simulink library "inp"  (Simulink 7.4)
settings: Solver=ode45  StartTime=0.0  StopTime=10.0  RelTol=1e-3
undefined symbols (not defined in the file): AINP_BrkPedalInterp_X_bar, C_TASK_10MS_S, ENUM_SHIFTER_D, ENUM_SHIFTER_N, ENUM_SHIFTER_P, ENUM_SHIFTER_R, KINP_BonnetCloseVehSpdThre_kph, KINP_EDUCoolantTempFilTm_s, KINP_EDUOilPressureFilTm_s, KINP_EDUOilTempFilTm_s, KINP_EDUSynchDisp_mm, KINP_EDUSynchPosnPWMDC_pct_LowerLimit, KINP_EDUSynchPosnPWMDC_pct_ovrdflg, KINP_EDUSynchPosnPWMDC_pct_ovrdval, KINP_EDUSynchPosnPWMDC_pct_UpperLimit, KINP_ShifterPosConfirmD_s, KINP_ShifterPosConfirmN_s, KINP_ShifterPosConfirmP_s, KINP_ShifterPosConfirmR_s, KINP_SingleAccPedalFltRateLim_pct, KINP_TMSpd2VehSpdSigNeg_rpm, KINP_TMSpd2VehSpdSigPos_rpm, KINP_ValidCheck_EDUSynchPosnPWMDC_dec, KINP_ValidCheck_EDUSynchPosnPWMDC_inc, KINP_ValidCheck_EDUSynchPosnPWMDC_lim, KINP_VehSpdSigKeepThres_kph, KPH2MPS, MIN2SEC, MINP_BrkPedalInterp_pct, MPS2KPH, PI, seat_version_control_block_callbacks, TIRE_RADIUS
libraries: inp_lib x166, hcu_lib x4, simulink x1
(part 8 of 9)

== system inp/INP/INP_50MS/BSRV_in_ovrdvals ==
  Constant: VSRV_AmbientTempIn_C_ovrdval : Constant  Value=0.0  OutDataTypeMode=single  OutDataTypeStr=single
  Constant: VSRV_AmbientTempValidIn_flg_ovrdval : Constant  Value=0  OutDataTypeMode=boolean  OutDataTypeStr=boolean
  Constant: VSRV_BMSCellTempMinIn_C_ovrdval : Constant  Value=0  OutDataTypeMode=boolean  OutDataTypeStr=boolean
  Constant: VSRV_BMSCellTempMinValidIn_flg_ovrdval : Constant  Value=0  OutDataTypeMode=boolean  OutDataTypeStr=boolean
  Constant: VSRV_BMSColdCrkCtrlIn_enum_ovrdval : Constant  Value=0  OutDataTypeMode=boolean  OutDataTypeStr=boolean
  Constant: VSRV_BMSHSC2FrP01Active_flg_ovrdval : Constant  Value=0  OutDataTypeMode=boolean  OutDataTypeStr=boolean
  Constant: VSRV_BMSHSC2FrP01ProtFault_flg_ovrdval : Constant  Value=0  OutDataTypeMode=boolean  OutDataTypeStr=boolean
  Constant: VSRV_BMSHSC2FrP02Active_flg_ovrdval : Constant  Value=0  OutDataTypeMode=boolean  OutDataTypeStr=boolean
  Constant: VSRV_BMSHSC2FrP02ProtFault_flg_ovrdval : Constant  Value=0  OutDataTypeMode=boolean  OutDataTypeStr=boolean
  Constant: VSRV_BMSMainRelayStatIn_enum_ovrdval : Constant  Value=0  OutDataTypeMode=uint8  OutDataTypeStr=uint8
  Constant: VSRV_BMSPackSOCDispIn_pct_ovrdval : Constant  Value=0  OutDataTypeMode=boolean  OutDataTypeStr=boolean
  Constant: VSRV_BMSPackSOCDispValidIn_pct_ovrdval : Constant  Value=0  OutDataTypeMode=boolean  OutDataTypeStr=boolean
  Constant: VSRV_HVBattBasicStatusIn_enum_ovrdval : Constant  Value=0  OutDataTypeMode=uint8  OutDataTypeStr=uint8
  Constant: VSRV_HVBattCellTempMaxIn_C_ovrdval : Constant  Value=0.0  OutDataTypeMode=single  OutDataTypeStr=single
  Constant: VSRV_HVBattCellTempMaxValidIn_flg_ovrdval : Constant  Value=0  OutDataTypeMode=boolean  OutDataTypeStr=boolean
  Constant: VSRV_HVBattChargerPluggedIn_flg_ovrdval : Constant  Value=0  OutDataTypeMode=boolean  OutDataTypeStr=boolean
  Constant: VSRV_HVBattChillerOffReqIn_flg_ovrdval : Constant  Value=0  OutDataTypeMode=boolean  OutDataTypeStr=boolean
  Constant: VSRV_HVBattCoolantTempIn_C_ovrdval : Constant  Value=0.0  OutDataTypeMode=single  OutDataTypeStr=single
  Constant: VSRV_HVBattCoolantTempValidIn_flg_ovrdval : Constant  Value=0  OutDataTypeMode=boolean  OutDataTypeStr=boolean
  Constant: VSRV_HVBattCoolingPumpStatusIn_enum_ovrdval : Constant  Value=0  OutDataTypeMode=uint8  OutDataTypeStr=uint8
  Constant: VSRV_HVBattCurrentIn_A_ovrdval : Constant  Value=0.0  OutDataTypeMode=single  OutDataTypeStr=single
  Constant: VSRV_HVBattCurrentValidIn_flg_ovrdval : Constant  Value=0  OutDataTypeMode=boolean  OutDataTypeStr=boolean
  Constant: VSRV_HVBattHVILClosedIn_flg_ovrdval : Constant  Value=0  OutDataTypeMode=boolean  OutDataTypeStr=boolean
  Constant: VSRV_HVBattIsolationResistanceIn_kohm_ovrdval : Constant  Value=0.0  OutDataTypeMode=single  OutDataTypeStr=single
  Constant: VSRV_HVBattIsolationResistanceValidIn_flg_ovrdval : Constant  Value=0  OutDataTypeMode=boolean  OutDataTypeStr=boolean
  Constant: VSRV_HVBattSOCIn_pct_ovrdval : Constant  Value=0.0  OutDataTypeMode=single  OutDataTypeStr=single
  Constant: VSRV_HVBattSOCValidIn_flg_ovrdval : Constant  Value=0  OutDataTypeMode=boolean  OutDataTypeStr=boolean
  Constant: VSRV_HVBattVoltageIn_V_ovrdval : Constant  Value=0.0  OutDataTypeMode=single  OutDataTypeStr=single
  Constant: VSRV_HVBattVoltageValidIn_flg_ovrdval : Constant  Value=0  OutDataTypeMode=boolean  OutDataTypeStr=boolean
  Constant: VSRV_KeySwitchStateCRKIn_flg_ovrdval : Constant  Value=0  OutDataTypeMode=boolean  OutDataTypeStr=boolean
  Constant: VSRV_SMUHSCFrP00Active_flg_ovrdval : Constant  Value=0  OutDataTypeMode=boolean  OutDataTypeStr=boolean
  Constant: VSRV_SMUHSCFrP03Active_flg_ovrdval : Constant  Value=0  OutDataTypeMode=boolean  OutDataTypeStr=boolean
  Constant: VSRV_SMUHSCFrP08Active_flg_ovrdval : Constant  Value=0  OutDataTypeMode=boolean  OutDataTypeStr=boolean
  inputs_bus : BusCreator  Inputs=33
  output_bus : Outport
  wires:
  Constant: VSRV_BMSPackSOCDispValidIn_pct_ovrdval/1 -> inputs_bus/33  "VSRV_BMSPackSOCDispValidIn_pct_ovrdval"
  Constant: VSRV_BMSPackSOCDispIn_pct_ovrdval/1 -> inputs_bus/32  "VSRV_BMSPackSOCDispIn_pct_ovrdval"
  Constant: VSRV_BMSCellTempMinValidIn_flg_ovrdval/1 -> inputs_bus/31  "VSRV_BMSCellTempMinValidIn_flg_ovrdval"
  Constant: VSRV_BMSCellTempMinIn_C_ovrdval/1 -> inputs_bus/30  "VSRV_BMSCellTempMinIn_C_ovrdval"
  Constant: VSRV_BMSColdCrkCtrlIn_enum_ovrdval/1 -> inputs_bus/29  "VSRV_BMSColdCrkCtrlIn_enum_ovrdval"
  Constant: VSRV_SMUHSCFrP00Active_flg_ovrdval/1 -> inputs_bus/28  "VSRV_SMUHSCFrP00Active_flg_ovrdval"
  Constant: VSRV_HVBattIsolationResistanceValidIn_flg_ovrdval/1 -> inputs_bus/27  "VSRV_HVBattIsolationResistanceValidIn_flg_ovrdval"
  Constant: VSRV_HVBattIsolationResistanceIn_kohm_ovrdval/1 -> inputs_bus/26  "VSRV_HVBattIsolationResistanceIn_kohm_ovrdval"
  Constant: VSRV_SMUHSCFrP08Active_flg_ovrdval/1 -> inputs_bus/25  "VSRV_SMUHSCFrP08Active_flg_ovrdval"
  Constant: VSRV_SMUHSCFrP03Active_flg_ovrdval/1 -> inputs_bus/24  "VSRV_SMUHSCFrP03Active_flg_ovrdval"
  Constant: VSRV_KeySwitchStateCRKIn_flg_ovrdval/1 -> inputs_bus/23  "VSRV_KeySwitchStateCRKIn_flg_ovrdval"
  Constant: VSRV_HVBattVoltageValidIn_flg_ovrdval/1 -> inputs_bus/22  "VSRV_HVBattVoltageValidIn_flg_ovrdval"
  Constant: VSRV_HVBattVoltageIn_V_ovrdval/1 -> inputs_bus/21  "VSRV_HVBattVoltageIn_V_ovrdval"
  Constant: VSRV_HVBattSOCValidIn_flg_ovrdval/1 -> inputs_bus/20  "VSRV_HVBattSOCValidIn_flg_ovrdval"
  Constant: VSRV_HVBattSOCIn_pct_ovrdval/1 -> inputs_bus/19  "VSRV_HVBattSOCIn_pct_ovrdval"
  Constant: VSRV_HVBattBasicStatusIn_enum_ovrdval/1 -> inputs_bus/18  "VSRV_HVBattBasicStatusIn_enum_ovrdval"
  Constant: VSRV_HVBattHVILClosedIn_flg_ovrdval/1 -> inputs_bus/17  "VSRV_HVBattHVILClosedIn_flg_ovrdval"
  Constant: VSRV_HVBattCurrentValidIn_flg_ovrdval/1 -> inputs_bus/16  "VSRV_HVBattCurrentValidIn_flg_ovrdval"
  Constant: VSRV_HVBattCurrentIn_A_ovrdval/1 -> inputs_bus/15  "VSRV_HVBattCurrentIn_A_ovrdval"
  Constant: VSRV_HVBattCoolingPumpStatusIn_enum_ovrdval/1 -> inputs_bus/14  "VSRV_HVBattCoolingPumpStatusIn_enum_ovrdval"
  Constant: VSRV_HVBattCoolantTempValidIn_flg_ovrdval/1 -> inputs_bus/13  "VSRV_HVBattCoolantTempValidIn_flg_ovrdval"
  Constant: VSRV_HVBattCoolantTempIn_C_ovrdval/1 -> inputs_bus/12  "VSRV_HVBattCoolantTempIn_C_ovrdval"
  Constant: VSRV_HVBattChillerOffReqIn_flg_ovrdval/1 -> inputs_bus/11  "VSRV_HVBattChillerOffReqIn_flg_ovrdval"
  Constant: VSRV_HVBattChargerPluggedIn_flg_ovrdval/1 -> inputs_bus/10  "VSRV_HVBattChargerPluggedIn_flg_ovrdval"
  Constant: VSRV_HVBattCellTempMaxValidIn_flg_ovrdval/1 -> inputs_bus/9  "VSRV_HVBattCellTempMaxValidIn_flg_ovrdval"
  Constant: VSRV_HVBattCellTempMaxIn_C_ovrdval/1 -> inputs_bus/8  "VSRV_HVBattCellTempMaxIn_C_ovrdval"
  Constant: VSRV_BMSMainRelayStatIn_enum_ovrdval/1 -> inputs_bus/7  "VSRV_BMSMainRelayStatIn_enum_ovrdval"
  Constant: VSRV_BMSHSC2FrP02Active_flg_ovrdval/1 -> inputs_bus/6  "VSRV_BMSHSC2FrP02Active_flg_ovrdval"
  Constant: VSRV_BMSHSC2FrP01Active_flg_ovrdval/1 -> inputs_bus/5  "VSRV_BMSHSC2FrP01Active_flg_ovrdval"
  Constant: VSRV_AmbientTempValidIn_flg_ovrdval/1 -> inputs_bus/4  "VSRV_AmbientTempValidIn_flg_ovrdval"
  Constant: VSRV_AmbientTempIn_C_ovrdval/1 -> inputs_bus/3  "VSRV_AmbientTempIn_C_ovrdval"
  Constant: VSRV_BMSHSC2FrP02ProtFault_flg_ovrdval/1 -> inputs_bus/2  "VSRV_BMSHSC2FrP02ProtFault_flg_ovrdval"
  Constant: VSRV_BMSHSC2FrP01ProtFault_flg_ovrdval/1 -> inputs_bus/1  "VSRV_BMSHSC2FrP01ProtFault_flg_ovrdval"
  inputs_bus/1 -> output_bus/1  "output_bus_ovrdval"

== system inp/INP/INP_50MS/Message (50ms) BMS_HSC2_FrP01 ==
  BHAL_IN_50ms : Inport
  BSRV_In_ovrdflgs : Inport  Port=2
  BSRV_In_ovrdvals : Inport  Port=3
  VINP_BMSMsgAlive_flg : Inport  Port=4
  Bus Creator : BusCreator  Inputs=5
  Bus Selector1 : BusSelector  OutputSignals=VHAL_HVBattSOCValidIn_flg
  Bus Selector11 : BusSelector  OutputSignals=VSRV_HVBattCurrentIn_A_ovrdval
  Bus Selector118 : BusSelector  OutputSignals=VHAL_HVBattSOCIn_pct
  Bus Selector120 : BusSelector  OutputSignals=VSRV_HVBattSOCIn_pct_ovrdflg
  Bus Selector142 : BusSelector  OutputSignals=VSRV_HVBattVoltageIn_V_ovrdflg
  Bus Selector143 : BusSelector  OutputSignals=VSRV_HVBattVoltageIn_V_ovrdval
  Bus Selector144 : BusSelector  OutputSignals=VHAL_HVBattVoltageIn_V
  Bus Selector15 : BusSelector  OutputSignals=VHAL_HVBattCurrentIn_A
  Bus Selector19 : BusSelector  OutputSignals=VSRV_HVBattCurrentIn_A_ovrdflg
  Bus Selector2 : BusSelector  OutputSignals=VSRV_BMSHSC2FrP01Active_flg_ovrdflg
  Bus Selector22 : BusSelector  OutputSignals=VHAL_HVBattCurrentValidIn_flg
  Bus Selector28 : BusSelector  OutputSignals=VSRV_HVBattSOCIn_pct_ovrdval
  Bus Selector3 : BusSelector  OutputSignals=VSRV_BMSHSC2FrP01Active_flg_ovrdval
  Bus Selector31 : BusSelector  OutputSignals=VSRV_HVBattIsolationResistanceIn_kohm_ovrdval
  Bus Selector32 : BusSelector  OutputSignals=VHAL_HVBattIsolationResistanceIn_kohm
  Bus Selector34 : BusSelector  OutputSignals=VSRV_HVBattIsolationResistanceIn_kohm_ovrdflg
  Bus Selector4 : BusSelector  OutputSignals=VHAL_HVBattVoltageValidIn_flg
  Bus Selector5 : BusSelector  OutputSignals=VHAL_HVBattIsolationResistanceValidIn_flg
  Subsys VINP_BMSHSC2FrP01Active_flg : inp_lib/override  SystemSampleTime=-1  cal_ovrdflg=KINP_BMSHSC2FrP01Active_ovrdflg  cal_ovrdval=KINP_BMSHSC2FrP01Active_flg_ovrdval
  Subsys VINP_HVBattCurrent_A : inp_lib/valid_msgactv_sat_ovrd  SystemSampleTime=-1  cal_ovrdflg=KINP_HVBattCurrent_A_ovrdflg  cal_ovrdval=KINP_HVBattCurrent_A_ovrdval  lim=KINP_ValidCheck_HVBattCurrent_lim  inc=KINP_ValidCheck_HVBattCurrent_inc  dec=KINP_ValidCheck_HVBattCurrent_dec  default=KINP_HVBattCurrentDefault_A  hi=KINP_HVBattCurrent_A_Max  lo=KINP_HVBattCurrent_A_Min
  Subsys VINP_HVBattIsolationResistance_kohm : inp_lib/valid_msgactv_sat_ovrd  SystemSampleTime=-1  cal_ovrdflg=KINP_HVBattIsolationResistance_kohm_ovrdflg  cal_ovrdval=KINP_HVBattIsolationResistance_kohm_ovrdval  lim=KINP_ValidCheck_HVBattIsolationResistance_lim  inc=KINP_ValidCheck_HVBattIsolationResistance_inc  dec=KINP_ValidCheck_HVBattIsolationResistance_dec  default=KINP_HVBattIsolationResistanceDefault_kohm  hi=KINP_HVBattIsolationResistance_kohm_Max  lo=KINP_HVBattIsolationResistance_kohm_Min
  Subsys VINP_HVBattSOC_pct : inp_lib/valid_msgactv_sat_ovrd  SystemSampleTime=-1  cal_ovrdflg=KINP_HVBattSOC_pct_ovrdflg  cal_ovrdval=KINP_HVBattSOC_pct_ovrdval  lim=KINP_ValidCheck_HVBattSOC_lim  inc=KINP_ValidCheck_HVBattSOC_inc  dec=KINP_ValidCheck_HVBattSOC_dec  default=KINP_HVBattSOCDefault_pct  hi=KINP_HVBattSOC_pct_Max  lo=KINP_HVBattSOC_pct_Min
  Subsys VINP_HVBattVoltage_V : inp_lib/valid_msgactv_sat_ovrd  SystemSampleTime=-1  cal_ovrdflg=KINP_HVBattVoltage_V_ovrdflg  cal_ovrdval=KINP_HVBattVoltage_V_ovrdval  lim=KINP_ValidCheck_HVBattVoltage_lim  inc=KINP_ValidCheck_HVBattVoltage_inc  dec=KINP_ValidCheck_HVBattVoltage_dec  default=KINP_HVBattVoltageDefault_V  hi=KINP_HVBattVoltage_V_Max  lo=KINP_HVBattVoltage_V_Min
  Terminator{,1..3} (4 alike) : Terminator
  BINP_BMS_FrP01 : Outport
  wires:
  [BSRV_In_ovrdvals] -> Bus Selector3/1
  [BSRV_In_ovrdflgs] -> Bus Selector2/1
  Bus Creator/1 -> BINP_BMS_FrP01/1  "BINP_BMS_FrP01"
  BSRV_In_ovrdvals/1 -> [BSRV_In_ovrdvals]
  BSRV_In_ovrdflgs/1 -> [BSRV_In_ovrdflgs]
  VINP_BMSMsgAlive_flg/1 -> [VINP_BMSMsgAlive_flg]
  [BSRV_In_ovrdflgs] -> Bus Selector120/1
  [BSRV_In_ovrdvals] -> Bus Selector28/1
  [BSRV_In_ovrdflgs] -> Bus Selector142/1
  [BSRV_In_ovrdvals] -> Bus Selector143/1
  [BSRV_In_ovrdflgs] -> Bus Selector19/1
  [BSRV_In_ovrdvals] -> Bus Selector11/1
  [BSRV_In_ovrdflgs] -> Bus Selector34/1
  [BSRV_In_ovrdvals] -> Bus Selector31/1
  BHAL_IN_50ms/1 -> Bus Selector32/1, Bus Selector5/1, Bus Selector118/1, Bus Selector1/1, Bus Selector4/1, Bus Selector22/1, Bus Selector15/1, Bus Selector144/1
  Bus Selector2/1 -> Subsys VINP_BMSHSC2FrP01Active_flg/2  "<VSRV_BMSHSC2FrP01Active_flg_ovrdflg>"
  Bus Selector3/1 -> Subsys VINP_BMSHSC2FrP01Active_flg/3  "<VSRV_BMSHSC2FrP01Active_flg_ovrdval>"
  Subsys VINP_BMSHSC2FrP01Active_flg/1 -> Bus Creator/5  "VINP_BMSHSC2FrP01Active_flg"
  Bus Selector15/1 -> Subsys VINP_HVBattCurrent_A/1  "<VHAL_HVBattCurrentIn_A>"
  Bus Selector22/1 -> Subsys VINP_HVBattCurrent_A/2  "<VHAL_HVBattCurrentValidIn_flg>"
  Bus Selector19/1 -> Subsys VINP_HVBattCurrent_A/3  "<VSRV_HVBattCurrentIn_A_ovrdflg>"
  Bus Selector11/1 -> Subsys VINP_HVBattCurrent_A/4  "<VSRV_HVBattCurrentIn_A_ovrdval>"
  [MsgAlive_flgs] -> Subsys VINP_HVBattCurrent_A/5
  Subsys VINP_HVBattCurrent_A/1 -> Bus Creator/4  "VINP_HVBattCurrent_A"
  Subsys VINP_HVBattCurrent_A/2 -> Terminator/1
  Bus Selector32/1 -> Subsys VINP_HVBattIsolationResistance_kohm/1  "<VHAL_HVBattIsolationResistanceIn_kohm>"
  Bus Selector5/1 -> Subsys VINP_HVBattIsolationResistance_kohm/2  "<VHAL_HVBattIsolationResistanceValidIn_flg>"
  Bus Selector34/1 -> Subsys VINP_HVBattIsolationResistance_kohm/3  "<VSRV_HVBattIsolationResistanceIn_kohm_ovrdflg>"
  Bus Selector31/1 -> Subsys VINP_HVBattIsolationResistance_kohm/4  "<VSRV_HVBattIsolationResistanceIn_kohm_ovrdval>"
  [MsgAlive_flgs] -> Subsys VINP_HVBattIsolationResistance_kohm/5
  Subsys VINP_HVBattIsolationResistance_kohm/1 -> Bus Creator/1  "VINP_HVBattIsolationResistance_kohm"
  Subsys VINP_HVBattIsolationResistance_kohm/2 -> Terminator1/1
  Bus Selector118/1 -> Subsys VINP_HVBattSOC_pct/1  "<VHAL_HVBattSOCIn_pct>"
  Bus Selector1/1 -> Subsys VINP_HVBattSOC_pct/2  "<VHAL_HVBattSOCValidIn_flg>"
  Bus Selector120/1 -> Subsys VINP_HVBattSOC_pct/3  "<VSRV_HVBattSOCIn_pct_ovrdflg>"
  Bus Selector28/1 -> Subsys VINP_HVBattSOC_pct/4  "<VSRV_HVBattSOCIn_pct_ovrdval>"
  [MsgAlive_flgs] -> Subsys VINP_HVBattSOC_pct/5
  Subsys VINP_HVBattSOC_pct/1 -> Bus Creator/2  "VINP_HVBattSOC_pct"
  Subsys VINP_HVBattSOC_pct/2 -> Terminator2/1
  Bus Selector144/1 -> Subsys VINP_HVBattVoltage_V/1  "<VHAL_HVBattVoltageIn_V>"
  Bus Selector4/1 -> Subsys VINP_HVBattVoltage_V/2  "<VHAL_HVBattVoltageValidIn_flg>"
  Bus Selector142/1 -> Subsys VINP_HVBattVoltage_V/3  "<VSRV_HVBattVoltageIn_V_ovrdflg>"
  Bus Selector143/1 -> Subsys VINP_HVBattVoltage_V/4  "<VSRV_HVBattVoltageIn_V_ovrdval>"
  [MsgAlive_flgs] -> Subsys VINP_HVBattVoltage_V/5
  Subsys VINP_HVBattVoltage_V/1 -> Bus Creator/3  "VINP_HVBattVoltage_V"
  Subsys VINP_HVBattVoltage_V/2 -> Terminator3/1
  [VINP_BMSMsgAlive_flg] -> Subsys VINP_BMSHSC2FrP01Active_flg/1, [MsgAlive_flgs]  "VINP_BMSMsgAlive_flg"

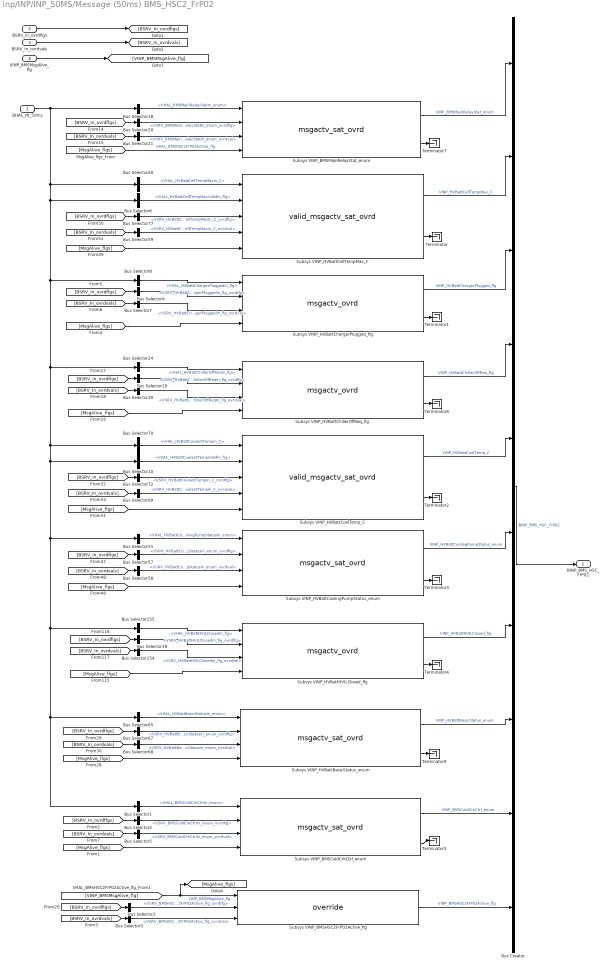
== system inp/INP/INP_50MS/Message (50ms) BMS_HSC2_FrP02 ==
  BHAL_IN_50ms : Inport
  BSRV_In_ovrdflgs : Inport  Port=2
  BSRV_In_ovrdvals : Inport  Port=3
  VINP_BMSMsgAlive_flg : Inport  Port=4
  Bus Creator : BusCreator  Inputs=10
  Bus Selector1 : BusSelector  OutputSignals=VHAL_BMSColdCrkCtrlIn_enum
  Bus Selector10 : BusSelector  OutputSignals=VHAL_HVBattCoolantTempValidIn_flg
  Bus Selector154 : BusSelector  OutputSignals=VSRV_HVBattHVILClosedIn_flg_ovrdval
  Bus Selector155 : BusSelector  OutputSignals=VHAL_HVBattHVILClosedIn_flg
  Bus Selector18 : BusSelector  OutputSignals=VHAL_BMSMainRelayStatIn_enum
  Bus Selector2 : BusSelector  OutputSignals=VSRV_BMSHSC2FrP02Active_flg_ovrdflg
  Bus Selector20 : BusSelector  OutputSignals=VSRV_BMSMainRelayStatIn_enum_ovrdflg
  Bus Selector21 : BusSelector  OutputSignals=VSRV_BMSMainRelayStatIn_enum_ovrdval
  Bus Selector24 : BusSelector  OutputSignals=VHAL_HVBattChillerOffReqIn_flg
  Bus Selector29 : BusSelector  OutputSignals=VSRV_HVBattChillerOffReqIn_flg_ovrdflg
  Bus Selector3 : BusSelector  OutputSignals=VSRV_BMSHSC2FrP02Active_flg_ovrdval
  Bus Selector30 : BusSelector  OutputSignals=VSRV_HVBattChillerOffReqIn_flg_ovrdval
  Bus Selector39 : BusSelector  OutputSignals=VSRV_HVBattHVILClosedIn_flg_ovrdflg
  Bus Selector4 : BusSelector  OutputSignals=VSRV_BMSColdCrkCtrlIn_enum_ovrdflg
  Bus Selector5 : BusSelector  OutputSignals=VSRV_BMSColdCrkCtrlIn_enum_ovrdval
  Bus Selector55 : BusSelector  OutputSignals=VHAL_HVBattCoolingPumpStatusIn_enum
  Bus Selector57 : BusSelector  OutputSignals=VSRV_HVBattCoolingPumpStatusIn_enum_ovrdflg
  Bus Selector58 : BusSelector  OutputSignals=VSRV_HVBattCoolingPumpStatusIn_enum_ovrdval
  Bus Selector59 : BusSelector  OutputSignals=VSRV_HVBattCellTempMaxIn_C_ovrdval
  Bus Selector6 : BusSelector  OutputSignals=VHAL_HVBattCellTempMaxValidIn_flg
  Bus Selector60 : BusSelector  OutputSignals=VHAL_HVBattCellTempMaxIn_C
  Bus Selector65 : BusSelector  OutputSignals=VHAL_HVBattBasicStatusIn_enum
  Bus Selector67 : BusSelector  OutputSignals=VSRV_HVBattBasicStatusIn_enum_ovrdflg
  Bus Selector68 : BusSelector  OutputSignals=VSRV_HVBattBasicStatusIn_enum_ovrdval
  Bus Selector69 : BusSelector  OutputSignals=VSRV_HVBattCoolantTempIn_C_ovrdval
  Bus Selector7 : BusSelector  OutputSignals=VSRV_HVBattChargerPluggedIn_flg_ovrdval
  Bus Selector70 : BusSelector  OutputSignals=VHAL_HVBattCoolantTempIn_C
  Bus Selector72 : BusSelector  OutputSignals=VSRV_HVBattCoolantTempIn_C_ovrdflg
  Bus Selector77 : BusSelector  OutputSignals=VSRV_HVBattCellTempMaxIn_C_ovrdflg
  Bus Selector8 : BusSelector  OutputSignals=VHAL_HVBattChargerPluggedIn_flg
  Bus Selector9 : BusSelector  OutputSignals=VSRV_HVBattChargerPluggedIn_flg_ovrdflg
  Subsys VINP_BMSColdCrkCtrl_enum : inp_lib/msgactv_sat_ovrd  SystemSampleTime=-1  cal_ovrdflg=KINP_BMSColdCrkCtrl_enum_ovrdflg  cal_ovrdval=KINP_BMSColdCrkCtrl_enum_ovrdval  default=KINP_BMSColdCrkCtrlDefault_enum  hi=KINP_BMSColdCrkCtrl_enum_Max  lo=KINP_BMSColdCrkCtrl_enum_Min
  Subsys VINP_BMSHSC2FrP02Active_flg : inp_lib/override  SystemSampleTime=-1  cal_ovrdflg=KINP_BMSHSC2FrP02Active_flg_ovrdflg  cal_ovrdval=KINP_BMSHSC2FrP02Active_flg_ovrdval
  Subsys VINP_BMSMainRelayStat_enum : inp_lib/msgactv_sat_ovrd  SystemSampleTime=-1  cal_ovrdflg=KINP_BMSMainRelayStat_enum_ovrdflg  cal_ovrdval=KINP_BMSMainRelayStat_enum_ovrdval  default=KINP_BMSMainRelayStatDefault_enum  hi=KINP_BMSMainRelayStat_enum_Max  lo=KINP_BMSMainRelayStat_enum_Min
  Subsys VINP_HVBattBasicStatus_enum : inp_lib/msgactv_sat_ovrd  SystemSampleTime=-1  cal_ovrdflg=KINP_HVBattBasicStatus_enum_ovrdflg  cal_ovrdval=KINP_HVBattBasicStatus_enum_ovrdval  default=KINP_HVBattBasicStatusDefault_enum  hi=KINP_HVBattBasicStatus_enum_Max  lo=KINP_HVBattBasicStatus_enum_Min
  Subsys VINP_HVBattCellTempMax_C : inp_lib/valid_msgactv_sat_ovrd  SystemSampleTime=-1  cal_ovrdflg=KINP_HVBattCellTempMax_C_ovrdflg  cal_ovrdval=KINP_HVBattCellTempMax_C_ovrdval  lim=KINP_ValidCheck_HVBattCellTempMax_lim  inc=KINP_ValidCheck_HVBattCellTempMax_inc  dec=KINP_ValidCheck_HVBattCellTempMax_dec  default=KINP_HVBattCellTempMaxDefault_C  hi=KINP_HVBattCellTempMax_C_Max  lo=KINP_HVBattCellTempMax_C_Min
  Subsys VINP_HVBattChargerPlugged_flg : inp_lib/msgactv_ovrd  SystemSampleTime=-1  cal_ovrdflg=KINP_HVBattChargerPlugged_flg_ovrdflg  cal_ovrdval=KINP_HVBattChargerPlugged_flg_ovrdval  default=KINP_HVBattChargerPluggedDefault_flg
  Subsys VINP_HVBattChillerOffReq_flg : inp_lib/msgactv_ovrd  SystemSampleTime=-1  cal_ovrdflg=KINP_HVBattChillerOffReq_flg_ovrdflg  cal_ovrdval=KINP_HVBattChillerOffReq_flg_ovrdval  default=KINP_HVBattChillerOffReqDefault_flg
  Subsys VINP_HVBattCoolTemp_C : inp_lib/valid_msgactv_sat_ovrd  SystemSampleTime=-1  cal_ovrdflg=KINP_HVBattCoolantTemp_C_ovrdflg  cal_ovrdval=KINP_HVBattCoolantTemp_C_ovrdval  lim=KINP_ValidCheck_HVBattCoolantTemp_lim  inc=KINP_ValidCheck_HVBattCoolantTemp_inc  dec=KINP_ValidCheck_HVBattCoolantTemp_dec  default=KINP_HVBattCoolantTempDefault_C  hi=KINP_HVBattCoolTemp_C_Max  lo=KINP_HVBattCoolTemp_C_Min
  Subsys VINP_HVBattCoolingPumpStatus_enum : inp_lib/msgactv_sat_ovrd  SystemSampleTime=-1  cal_ovrdflg=KINP_HVBattCoolingPumpStatus_enum_ovrdflg  cal_ovrdval=KINP_HVBattCoolingPumpStatus_enum_ovrdval  default=KINP_HVBattCoolingPumpStatusDefault_enum  hi=KINP_HVBattCoolingPumpStatus_enum_Max  lo=KINP_HVBattCoolingPumpStatus_enum_Min
  Subsys VINP_HVBattHVILClosed_flg : inp_lib/msgactv_ovrd  SystemSampleTime=-1  cal_ovrdflg=KINP_HVBattHVILClosed_flg_ovrdflg  cal_ovrdval=KINP_HVBattHVILClosed_flg_ovrdval  default=KINP_HVBattHVILClosedDefault_flg
  Terminator{,1..5,7..9} (9 alike) : Terminator
  BINP_BMS_HSC_FrP02 : Outport
  wires:
  Subsys VINP_BMSHSC2FrP02Active_flg/1 -> Bus Creator/10  "VINP_BMSHSC2FrP02Active_flg"
  [BSRV_In_ovrdflgs] -> Bus Selector4/1
  [BSRV_In_ovrdvals] -> Bus Selector5/1
  Bus Selector1/1 -> Subsys VINP_BMSColdCrkCtrl_enum/1  "<VHAL_BMSColdCrkCtrlIn_enum>"
  Bus Selector4/1 -> Subsys VINP_BMSColdCrkCtrl_enum/2  "<VSRV_BMSColdCrkCtrlIn_enum_ovrdflg>"
  Bus Selector5/1 -> Subsys VINP_BMSColdCrkCtrl_enum/3  "<VSRV_BMSColdCrkCtrlIn_enum_ovrdval>"
  [MsgAlive_flgs] -> Subsys VINP_BMSColdCrkCtrl_enum/4
  Subsys VINP_BMSColdCrkCtrl_enum/1 -> Bus Creator/9  "VINP_BMSColdCrkCtrl_enum"
  Subsys VINP_BMSColdCrkCtrl_enum/2 -> Terminator5/1
  BHAL_IN_50ms/1 -> Bus Selector60/1, Bus Selector6/1, Bus Selector8/1, Bus Selector24/1, Bus Selector70/1, Bus Selector10/1, Bus Selector55/1, Bus Selector1/1, Bus Selector65/1, Bus Selector155/1, Bus Selector18/1
  [BSRV_In_ovrdvals] -> Bus Selector21/1
  [BSRV_In_ovrdflgs] -> Bus Selector20/1
  VINP_BMSMsgAlive_flg/1 -> [VINP_BMSMsgAlive_flg]
  BSRV_In_ovrdflgs/1 -> [BSRV_In_ovrdflgs]
  BSRV_In_ovrdvals/1 -> [BSRV_In_ovrdvals]
  Bus Creator/1 -> BINP_BMS_HSC_FrP02/1  "BINP_BMS_HSC_FrP02"
  [BSRV_In_ovrdflgs] -> Bus Selector77/1
  [BSRV_In_ovrdvals] -> Bus Selector59/1
  [BSRV_In_ovrdflgs] -> Bus Selector9/1
  [BSRV_In_ovrdvals] -> Bus Selector7/1
  [BSRV_In_ovrdflgs] -> Bus Selector29/1
  [BSRV_In_ovrdvals] -> Bus Selector30/1
  [BSRV_In_ovrdflgs] -> Bus Selector72/1
  [BSRV_In_ovrdvals] -> Bus Selector69/1
  [BSRV_In_ovrdflgs] -> Bus Selector57/1
  [BSRV_In_ovrdvals] -> Bus Selector58/1
  [BSRV_In_ovrdflgs] -> Bus Selector39/1
  [BSRV_In_ovrdvals] -> Bus Selector154/1
  [BSRV_In_ovrdflgs] -> Bus Selector67/1
  [BSRV_In_ovrdvals] -> Bus Selector68/1
  [BSRV_In_ovrdvals] -> Bus Selector3/1
  [BSRV_In_ovrdflgs] -> Bus Selector2/1
  Bus Selector2/1 -> Subsys VINP_BMSHSC2FrP02Active_flg/2  "<VSRV_BMSHSC2FrP02Active_flg_ovrdflg>"
  Bus Selector3/1 -> Subsys VINP_BMSHSC2FrP02Active_flg/3  "<VSRV_BMSHSC2FrP02Active_flg_ovrdval>"
  Bus Selector60/1 -> Subsys VINP_HVBattCellTempMax_C/1  "<VHAL_HVBattCellTempMaxIn_C>"
  Bus Selector6/1 -> Subsys VINP_HVBattCellTempMax_C/2  "<VHAL_HVBattCellTempMaxValidIn_flg>"
  Bus Selector77/1 -> Subsys VINP_HVBattCellTempMax_C/3  "<VSRV_HVBattCellTempMaxIn_C_ovrdflg>"
  Bus Selector59/1 -> Subsys VINP_HVBattCellTempMax_C/4  "<VSRV_HVBattCellTempMaxIn_C_ovrdval>"
  [MsgAlive_flgs] -> Subsys VINP_HVBattCellTempMax_C/5
  Subsys VINP_HVBattCellTempMax_C/1 -> Bus Creator/2  "VINP_HVBattCellTempMax_C"
  Subsys VINP_HVBattCellTempMax_C/2 -> Terminator/1
  Bus Selector8/1 -> Subsys VINP_HVBattChargerPlugged_flg/1  "<VHAL_HVBattChargerPluggedIn_flg>"
  Bus Selector9/1 -> Subsys VINP_HVBattChargerPlugged_flg/2  "<VSRV_HVBattChargerPluggedIn_flg_ovrdflg>"
  Bus Selector7/1 -> Subsys VINP_HVBattChargerPlugged_flg/3  "<VSRV_HVBattChargerPluggedIn_flg_ovrdval>"
  [MsgAlive_flgs] -> Subsys VINP_HVBattChargerPlugged_flg/4
  Subsys VINP_HVBattChargerPlugged_flg/1 -> Bus Creator/3  "VINP_HVBattChargerPlugged_flg"
  Subsys VINP_HVBattChargerPlugged_flg/2 -> Terminator1/1
  Bus Selector70/1 -> Subsys VINP_HVBattCoolTemp_C/1  "<VHAL_HVBattCoolantTempIn_C>"
  Bus Selector10/1 -> Subsys VINP_HVBattCoolTemp_C/2  "<VHAL_HVBattCoolantTempValidIn_flg>"
  Bus Selector72/1 -> Subsys VINP_HVBattCoolTemp_C/3  "<VSRV_HVBattCoolantTempIn_C_ovrdflg>"
  Bus Selector69/1 -> Subsys VINP_HVBattCoolTemp_C/4  "<VSRV_HVBattCoolantTempIn_C_ovrdval>"
  [MsgAlive_flgs] -> Subsys VINP_HVBattCoolTemp_C/5
  Subsys VINP_HVBattCoolTemp_C/1 -> Bus Creator/5  "VINP_HVBattCoolTemp_C"
  Subsys VINP_HVBattCoolTemp_C/2 -> Terminator2/1
  Bus Selector55/1 -> Subsys VINP_HVBattCoolingPumpStatus_enum/1  "<VHAL_HVBattCoolingPumpStatusIn_enum>"
  Bus Selector57/1 -> Subsys VINP_HVBattCoolingPumpStatus_enum/2  "<VSRV_HVBattCoolingPumpStatusIn_enum_ovrdflg>"
  Bus Selector58/1 -> Subsys VINP_HVBattCoolingPumpStatus_enum/3  "<VSRV_HVBattCoolingPumpStatusIn_enum_ovrdval>"
  [MsgAlive_flgs] -> Subsys VINP_HVBattCoolingPumpStatus_enum/4
  Subsys VINP_HVBattCoolingPumpStatus_enum/1 -> Bus Creator/6  "VINP_HVBattCoolingPumpStatus_enum"
  Subsys VINP_HVBattCoolingPumpStatus_enum/2 -> Terminator3/1
  Bus Selector155/1 -> Subsys VINP_HVBattHVILClosed_flg/1  "<VHAL_HVBattHVILClosedIn_flg>"
  Bus Selector39/1 -> Subsys VINP_HVBattHVILClosed_flg/2  "<VSRV_HVBattHVILClosedIn_flg_ovrdflg>"
  Bus Selector154/1 -> Subsys VINP_HVBattHVILClosed_flg/3  "<VSRV_HVBattHVILClosedIn_flg_ovrdval>"
  [MsgAlive_flgs] -> Subsys VINP_HVBattHVILClosed_flg/4
  Subsys VINP_HVBattHVILClosed_flg/1 -> Bus Creator/7  "VINP_HVBattHVILClosed_flg"
  Subsys VINP_HVBattHVILClosed_flg/2 -> Terminator4/1
  Bus Selector18/1 -> Subsys VINP_BMSMainRelayStat_enum/1  "<VHAL_BMSMainRelayStatIn_enum>"
  Bus Selector20/1 -> Subsys VINP_BMSMainRelayStat_enum/2  "<VSRV_BMSMainRelayStatIn_enum_ovrdflg>"
  Bus Selector21/1 -> Subsys VINP_BMSMainRelayStat_enum/3  "<VSRV_BMSMainRelayStatIn_enum_ovrdval>"
  [MsgAlive_flgs] -> Subsys VINP_BMSMainRelayStat_enum/4  "VHAL_BMSHSC2FrP02Active_flg"
  Subsys VINP_BMSMainRelayStat_enum/1 -> Bus Creator/1  "VINP_BMSMainRelayStat_enum"
  Subsys VINP_BMSMainRelayStat_enum/2 -> Terminator7/1
  Bus Selector24/1 -> Subsys VINP_HVBattChillerOffReq_flg/1  "<VHAL_HVBattChillerOffReqIn_flg>"
  Bus Selector29/1 -> Subsys VINP_HVBattChillerOffReq_flg/2  "<VSRV_HVBattChillerOffReqIn_flg_ovrdflg>"
  Bus Selector30/1 -> Subsys VINP_HVBattChillerOffReq_flg/3  "<VSRV_HVBattChillerOffReqIn_flg_ovrdval>"
  [MsgAlive_flgs] -> Subsys VINP_HVBattChillerOffReq_flg/4
  Subsys VINP_HVBattChillerOffReq_flg/1 -> Bus Creator/4  "VINP_HVBattChillerOffReq_flg"
  Subsys VINP_HVBattChillerOffReq_flg/2 -> Terminator8/1
  Bus Selector65/1 -> Subsys VINP_HVBattBasicStatus_enum/1  "<VHAL_HVBattBasicStatusIn_enum>"
  Bus Selector67/1 -> Subsys VINP_HVBattBasicStatus_enum/2  "<VSRV_HVBattBasicStatusIn_enum_ovrdflg>"
  Bus Selector68/1 -> Subsys VINP_HVBattBasicStatus_enum/3  "<VSRV_HVBattBasicStatusIn_enum_ovrdval>"
  [MsgAlive_flgs] -> Subsys VINP_HVBattBasicStatus_enum/4
  Subsys VINP_HVBattBasicStatus_enum/1 -> Bus Creator/8  "VINP_HVBattBasicStatus_enum"
  Subsys VINP_HVBattBasicStatus_enum/2 -> Terminator9/1
  [VINP_BMSMsgAlive_flg] -> Subsys VINP_BMSHSC2FrP02Active_flg/1, [MsgAlive_flgs]  "VINP_BMSMsgAlive_flg"

== system inp/INP/INP_50MS/Message (50ms) BMS_HSC2_FrP05 ==
  BHAL_IN_50ms : Inport
  BSRV_In_ovrdflgs : Inport  Port=2
  BSRV_In_ovrdvals : Inport  Port=3
  VINP_BMSMsgAlive_flg : Inport  Port=4
  Bus Creator : BusCreator  Inputs=2
  Bus Selector1 : BusSelector  OutputSignals=VHAL_BMSPackSOCDispValidIn_flg
  Bus Selector118 : BusSelector  OutputSignals=VHAL_BMSPackSOCDispIn_pct
  Bus Selector120 : BusSelector  OutputSignals=VSRV_BMSPackSOCDispIn_pct_ovrdflg
  Bus Selector28 : BusSelector  OutputSignals=VSRV_BMSPackSOCDispValidIn_pct_ovrdval
  Bus Selector59 : BusSelector  OutputSignals=VSRV_BMSCellTempMinIn_C_ovrdval
  Bus Selector6 : BusSelector  OutputSignals=VHAL_BMSCellTempMinValidIn_flg
  Bus Selector60 : BusSelector  OutputSignals=VHAL_BMSCellTempMinIn_C
  Bus Selector77 : BusSelector  OutputSignals=VSRV_BMSCellTempMinIn_C_ovrdflg
  Subsys VINP_BMSCellTempMin_C : inp_lib/valid_msgactv_sat_ovrd  SystemSampleTime=-1  cal_ovrdflg=KINP_BMSCellTempMin_C_ovrdflg  cal_ovrdval=KINP_BMSCellTempMin_C_ovrdval  lim=KINP_ValidCheck_BMSCellTempMin_lim  inc=KINP_ValidCheck_BMSCellTempMin_inc  dec=KINP_ValidCheck_BMSCellTempMin_dec  default=KINP_BMSCellTempMinDefault_C  hi=KINP_BMSCellTempMin_C_Max  lo=KINP_BMSCellTempMin_C_Min
  Subsys VINP_BMSPackSOCDisp_pct : inp_lib/valid_msgactv_sat_ovrd  SystemSampleTime=-1  cal_ovrdflg=KINP_BMSPackSOCDisp_pct_ovrdflg  cal_ovrdval=KINP_BMSPackSOCDisp_pct_ovrdval  lim=KINP_ValidCheck_BMSPackSOCDisp_lim  inc=KINP_ValidCheck_BMSPackSOCDisp_inc  dec=KINP_ValidCheck_BMSPackSOCDisp_dec  default=KINP_BMSPackSOCDispDefault_pct  hi=KINP_BMSPackSOCDisp_pct_Max  lo=KINP_BMSPackSOCDisp_pct_Min
  Terminator : Terminator
  Terminator2 : Terminator
  BINP_BMS_HSC_FrP05 : Outport
  wires:
  Subsys VINP_BMSCellTempMin_C/1 -> Bus Creator/1  "VINP_BMSCellTempMin_C"
  [BSRV_In_ovrdflgs] -> Bus Selector120/1
  [BSRV_In_ovrdvals] -> Bus Selector28/1
  Bus Selector118/1 -> Subsys VINP_BMSPackSOCDisp_pct/1  "<VHAL_BMSPackSOCDispIn_pct>"
  Bus Selector1/1 -> Subsys VINP_BMSPackSOCDisp_pct/2  "<VHAL_BMSPackSOCDispValidIn_flg>"
  Bus Selector120/1 -> Subsys VINP_BMSPackSOCDisp_pct/3  "<VSRV_BMSPackSOCDispIn_pct_ovrdflg>"
  Bus Selector28/1 -> Subsys VINP_BMSPackSOCDisp_pct/4  "<VSRV_BMSPackSOCDispValidIn_pct_ovrdval>"
  [MsgAlive_flgs] -> Subsys VINP_BMSPackSOCDisp_pct/5
  Subsys VINP_BMSPackSOCDisp_pct/1 -> Bus Creator/2  "VINP_BMSPackSOCDisp_pct"
  Subsys VINP_BMSPackSOCDisp_pct/2 -> Terminator2/1
  BHAL_IN_50ms/1 -> Bus Selector1/1, Bus Selector118/1, Bus Selector6/1, Bus Selector60/1
  VINP_BMSMsgAlive_flg/1 -> [MsgAlive_flgs]
  BSRV_In_ovrdflgs/1 -> [BSRV_In_ovrdflgs]
  BSRV_In_ovrdvals/1 -> [BSRV_In_ovrdvals]
  Bus Creator/1 -> BINP_BMS_HSC_FrP05/1  "BINP_BMS_HSC_FrP05"
  [BSRV_In_ovrdflgs] -> Bus Selector77/1
  [BSRV_In_ovrdvals] -> Bus Selector59/1
  Bus Selector60/1 -> Subsys VINP_BMSCellTempMin_C/1  "<VHAL_BMSCellTempMinIn_C>"
  Bus Selector6/1 -> Subsys VINP_BMSCellTempMin_C/2  "<VHAL_BMSCellTempMinValidIn_flg>"
  Bus Selector77/1 -> Subsys VINP_BMSCellTempMin_C/3  "<VSRV_BMSCellTempMinIn_C_ovrdflg>"
  Bus Selector59/1 -> Subsys VINP_BMSCellTempMin_C/4  "<VSRV_BMSCellTempMinIn_C_ovrdval>"
  [MsgAlive_flgs] -> Subsys VINP_BMSCellTempMin_C/5
  Subsys VINP_BMSCellTempMin_C/2 -> Terminator/1

== system inp/INP/INP_50MS/Message (50ms) SMU_HSC_FrP03 ==
  BHAL_IN_50ms : Inport
  BSRV_In_ovrdflgs : Inport  Port=2
  BSRV_In_ovrdvals : Inport  Port=3
  VINP_SMUMsgAlive_flg : Inport  Port=4
  Bus Creator : BusCreator  Inputs=3
  Bus Selector1 : BusSelector  OutputSignals=VHAL_AmbientTempIn_C
  Bus Selector2 : BusSelector  OutputSignals=VSRV_SMUHSCFrP03Active_flg_ovrdflg
  Bus Selector20 : BusSelector  OutputSignals=VSRV_AmbientTempIn_C_ovrdflg
  Bus Selector23 : BusSelector  OutputSignals=VSRV_AmbientTempIn_C_ovrdval
  Bus Selector3 : BusSelector  OutputSignals=VSRV_SMUHSCFrP03Active_flg_ovrdval
  Bus Selector4 : BusSelector  OutputSignals=VHAL_AmbientTempValidIn_flg
  Bus Selector5 : BusSelector  OutputSignals=VSRV_KeySwitchStateCRKIn_flg_ovrdflg
  Bus Selector6 : BusSelector  OutputSignals=VSRV_KeySwitchStateCRKIn_flg_ovrdval
  Bus Selector7 : BusSelector  OutputSignals=VHAL_KeySwitchStateCRKIn_flg
  Subsys VINP_AmbientTemp_C : inp_lib/valid_msgactv_sat_ovrd  SystemSampleTime=-1  cal_ovrdflg=KINP_AmbientTemp_C_ovrdflg  cal_ovrdval=KINP_AmbientTemp_C_ovrdval  lim=KINP_ValidCheck_AmbientTemp_lim  inc=KINP_ValidCheck_AmbientTemp_inc  dec=KINP_ValidCheck_AmbientTemp_dec  default=KINP_AmbientTempDefault_C  hi=KINP_AmbientTemp_C_Max  lo=KINP_AmbientTemp_C_Min
  Subsys VINP_KeySwitchStateCRK_flg : inp_lib/msgactv_ovrd  SystemSampleTime=-1  cal_ovrdflg=KINP_KeySwitchStateCRK_flg_ovrdflg  cal_ovrdval=KINP_KeySwitchStateCRK_flg_ovrdval  default=KINP_KeySwitchStateCRKDefault_flg
  Subsys VINP_SMUHSCFrP03Active_flg : inp_lib/override  SystemSampleTime=-1  cal_ovrdflg=KINP_SMUHSCFrP03Active_ovrdflg  cal_ovrdval=KINP_SMUHSCFrP03Active_flg_ovrdval
  Terminator : Terminator
  Terminator1 : Terminator
  BINP_SMU_HSC_FrP03 : Outport
  wires:
  [BSRV_In_ovrdvals] -> Bus Selector3/1
  [BSRV_In_ovrdflgs] -> Bus Selector2/1
  [VINP_SMUMsgAlive_flg] -> [MsgAlive_flgs], Subsys VINP_SMUHSCFrP03Active_flg/1
  VINP_SMUMsgAlive_flg/1 -> [VINP_SMUMsgAlive_flg]
  BSRV_In_ovrdflgs/1 -> [BSRV_In_ovrdflgs]
  BSRV_In_ovrdvals/1 -> [BSRV_In_ovrdvals]
  [BSRV_In_ovrdvals] -> Bus Selector23/1
  [BSRV_In_ovrdflgs] -> Bus Selector20/1
  BHAL_IN_50ms/1 -> Bus Selector1/1, Bus Selector4/1, Bus Selector7/1
  [BSRV_In_ovrdvals] -> Bus Selector6/1
  [BSRV_In_ovrdflgs] -> Bus Selector5/1
  Bus Creator/1 -> BINP_SMU_HSC_FrP03/1  "BINP_SMU_HSC_FrP03"
  Bus Selector1/1 -> Subsys VINP_AmbientTemp_C/1  "<VHAL_AmbientTempIn_C>"
  Bus Selector4/1 -> Subsys VINP_AmbientTemp_C/2  "<VHAL_AmbientTempValidIn_flg>"
  Bus Selector20/1 -> Subsys VINP_AmbientTemp_C/3  "<VSRV_AmbientTempIn_C_ovrdflg>"
  Bus Selector23/1 -> Subsys VINP_AmbientTemp_C/4  "<VSRV_AmbientTempIn_C_ovrdval>"
  [MsgAlive_flgs] -> Subsys VINP_AmbientTemp_C/5
  Subsys VINP_AmbientTemp_C/1 -> Bus Creator/1  "VINP_AmbientTemp_C"
  Subsys VINP_AmbientTemp_C/2 -> Terminator/1
  Bus Selector7/1 -> Subsys VINP_KeySwitchStateCRK_flg/1  "<VHAL_KeySwitchStateCRKIn_flg>"
  Bus Selector5/1 -> Subsys VINP_KeySwitchStateCRK_flg/2  "<VSRV_KeySwitchStateCRKIn_flg_ovrdflg>"
  Bus Selector6/1 -> Subsys VINP_KeySwitchStateCRK_flg/3  "<VSRV_KeySwitchStateCRKIn_flg_ovrdval>"
  [MsgAlive_flgs] -> Subsys VINP_KeySwitchStateCRK_flg/4
  Subsys VINP_KeySwitchStateCRK_flg/1 -> Bus Creator/2  "VINP_KeySwitchStateCRK_flg"
  Subsys VINP_KeySwitchStateCRK_flg/2 -> Terminator1/1
  Bus Selector2/1 -> Subsys VINP_SMUHSCFrP03Active_flg/2  "<VSRV_SMUHSCFrP03Active_flg_ovrdflg>"
  Bus Selector3/1 -> Subsys VINP_SMUHSCFrP03Active_flg/3  "<VSRV_SMUHSCFrP03Active_flg_ovrdval>"
  Subsys VINP_SMUHSCFrP03Active_flg/1 -> Bus Creator/3  "VINP_SMUHSCFrP03Active_flg"

== system inp/INP/INP_5MS/BSRV_In_ovrdflgs ==
  Constant: VSRV_EDUOutputShaftSpdRawIn_rpm_ovrdflg : Constant  Value=0  OutDataTypeMode=boolean  OutDataTypeStr=boolean
  Constant: VSRV_EDUOutputShaftSpdRawValidIn_flg_ovrdflg : Constant  Value=0  OutDataTypeMode=boolean  OutDataTypeStr=boolean
  Constant: VSRV_EDUSynchPosnIn_mm_ovrdflg : Constant  Value=0  OutDataTypeMode=boolean  OutDataTypeStr=boolean
  Constant: VSRV_EDUSynchPosnPWMDCValidIn_flg_ovrdflg : Constant  Value=0  OutDataTypeMode=boolean  OutDataTypeStr=boolean
  Constant: VSRV_EDUSynchPosnPWMKDCIn_pct_ovrdflg : Constant  Value=0  OutDataTypeMode=boolean  OutDataTypeStr=boolean
  Constant: VSRV_EDUSynchPosnPWMKDCValidIn_flg_ovrdflg : Constant  Value=0  OutDataTypeMode=boolean  OutDataTypeStr=boolean
  inputs_bus : BusCreator  Inputs=6
  output_bus : Outport
  wires:
  Constant: VSRV_EDUOutputShaftSpdRawValidIn_flg_ovrdflg/1 -> inputs_bus/6  "VSRV_EDUOutputShaftSpdRawValidIn_flg_ovrdflg"
  Constant: VSRV_EDUOutputShaftSpdRawIn_rpm_ovrdflg/1 -> inputs_bus/5  "VSRV_EDUOutputShaftSpdRawIn_rpm_ovrdflg"
  Constant: VSRV_EDUSynchPosnPWMDCValidIn_flg_ovrdflg/1 -> inputs_bus/4  "VSRV_EDUSynchPosnPWMDCValidIn_flg_ovrdflg"
  Constant: VSRV_EDUSynchPosnIn_mm_ovrdflg/1 -> inputs_bus/3  "VSRV_EDUSynchPosnPWMDCIn_pct_ovrdflg"
  Constant: VSRV_EDUSynchPosnPWMKDCValidIn_flg_ovrdflg/1 -> inputs_bus/2  "VSRV_EDUSynchPosnPWMKDCValidIn_flg_ovrdflg"
  Constant: VSRV_EDUSynchPosnPWMKDCIn_pct_ovrdflg/1 -> inputs_bus/1  "VSRV_EDUSynchPosnPWMKDCIn_pct_ovrdflg"
  inputs_bus/1 -> output_bus/1  "output_bus"

== system inp/INP/INP_5MS/BSRV_in_ovrdvals ==
  Constant: VSRV_EDUOutputShaftSpdRawIn_rpm_ovrdval : Constant  Value=0.0  OutDataTypeMode=single  OutDataTypeStr=single
  Constant: VSRV_EDUOutputShaftSpdRawValidIn_flg_ovrdval : Constant  Value=0  OutDataTypeMode=boolean  OutDataTypeStr=boolean
  Constant: VSRV_EDUSynchPosnPWMDCIn_pct_ovrdval : Constant  Value=0.0  OutDataTypeMode=single  OutDataTypeStr=single
  Constant: VSRV_EDUSynchPosnPWMDCValidIn_flg_ovrdflg : Constant  Value=0  OutDataTypeMode=boolean  OutDataTypeStr=boolean
  Constant: VSRV_EDUSynchPosnPWMKDCIn_pct_ovrdval : Constant  Value=0.0  OutDataTypeMode=single  OutDataTypeStr=single
  Constant:VSRV_EDUSynchPosnPWMKDCValidIn_flg_ovrdval : Constant  Value=0  OutDataTypeMode=boolean  OutDataTypeStr=boolean
  inputs_bus : BusCreator  Inputs=6
  output_bus : Outport
  wires:
  Constant: VSRV_EDUOutputShaftSpdRawValidIn_flg_ovrdval/1 -> inputs_bus/6  "VSRV_EDUOutputShaftSpdRawValidIn_flg_ovrdval"
  Constant: VSRV_EDUOutputShaftSpdRawIn_rpm_ovrdval/1 -> inputs_bus/5  "VSRV_EDUOutputShaftSpdRawIn_rpm_ovrdval"
  Constant: VSRV_EDUSynchPosnPWMDCValidIn_flg_ovrdflg/1 -> inputs_bus/4  "VSRV_EDUSynchPosnPWMDCValidIn_flg_ovrdflg"
  Constant: VSRV_EDUSynchPosnPWMDCIn_pct_ovrdval/1 -> inputs_bus/3  "VSRV_EDUSynchPosnPWMDCIn_pct_ovrdval"
  Constant:VSRV_EDUSynchPosnPWMKDCValidIn_flg_ovrdval/1 -> inputs_bus/2  "VSRV_EDUSynchPosnPWMKDCValidIn_flg_ovrdval"
  Constant: VSRV_EDUSynchPosnPWMKDCIn_pct_ovrdval/1 -> inputs_bus/1  "VSRV_EDUSynchPosnPWMKDCIn_pct_ovrdval"
  inputs_bus/1 -> output_bus/1  "output_bus_ovrdval"

== system inp/INP/INP_5MS/HW_HCU_5ms ==
  BHAL_outputs : Inport  OutDataType=sfix(16)  OutScaling=2^0
  BSRV_In_ovrdflgs : Inport  Port=2  OutDataType=sfix(16)  OutScaling=2^0
  BSRV_In_ovrdvals : Inport  Port=3  OutDataType=sfix(16)  OutScaling=2^0
  Bus Creator1 : BusCreator  Inputs=6
  Bus Selector17 : BusSelector  OutputSignals=VSRV_EDUSynchPosnPWMKDCIn_pct_ovrdval
  Bus Selector18 : BusSelector  OutputSignals=VSRV_EDUSynchPosnPWMKDCIn_pct_ovrdflg
  Bus Selector19 : BusSelector  OutputSignals=VHAL_EDUSynchPosnPWMKDCIn_pct
  Bus Selector22 : BusSelector  OutputSignals=VSRV_EDUOutputShaftSpdRawIn_rpm_ovrdval
  Bus Selector23 : BusSelector  OutputSignals=VSRV_EDUOutputShaftSpdRawIn_rpm_ovrdflg
  Bus Selector24 : BusSelector  OutputSignals=VHAL_EDUOutputShaftSpdRawIn_rpm
  Bus Selector28 : BusSelector  OutputSignals=VSRV_EDUSynchPosnPWMDCIn_pct_ovrdval
  Bus Selector29 : BusSelector  OutputSignals=VSRV_EDUSynchPosnPWMDCIn_pct_ovrdflg
  Bus Selector30 : BusSelector  OutputSignals=VHAL_EDUSynchPosnPWMDCIn_pct
  Bus Selector41 : BusSelector  OutputSignals=VHAL_EDUOutputShaftSpdRawValidIn_flg
  Bus Selector43 : BusSelector  OutputSignals=VHAL_EDUSynchPosnPWMDCValidIn_flg
  Bus Selector50 : BusSelector  OutputSignals=VHAL_EDUSynchPosnPWMKDCValidIn_flg
  Subsys VINP_EDUOutputShaftSpdRaw_rpm : inp_lib/valid_sat_ovrd  SystemSampleTime=-1  cal_ovrdflg=KINP_EDUOutputShaftSpdRaw_rpm_ovrdflg  cal_ovrdval=KINP_EDUOutputShaftSpdRaw_rpm_ovrdval  lim=KINP_ValidCheck_EDUOutputShaftSpdRaw_lim  inc=KINP_ValidCheck_EDUOutputShaftSpdRaw_inc  dec=KINP_ValidCheck_EDUOutputShaftSpdRaw_dec  default=KINP_EDUOutputShaftSpdRawDefault_rpm  hi=KINP_EDUOutputShaftSpdRaw_rpm_UpperLimit  lo=KINP_EDUOutputShaftSpdRaw_rpm_LowerLimit
  Subsys VINP_EDUSynchPosnPWMDC_pct : Subsystem  mask{cal_ovrdflg=KINP_EDUSynchPosnPWMDC_pct_ovrdflg, cal_ovrdval=KINP_EDUSynchPosnPWMDC_pct_ovrdval, lim=KINP_ValidCheck_EDUSynchPosnPWMDC_lim, inc=KINP_ValidCheck_EDUSynchPosnPWMDC_inc, dec=KINP_ValidCheck_EDUSynchPosnPWMDC_dec, default=0, hi=KINP_EDUSynchPosnPWMDC_pct_UpperLimit, lo=KINP_EDUSynchPosnPWMDC_pct_LowerLimit}
      mask prompts: cal_ovrdflg "Override Flag"; cal_ovrdval "Override Value"; lim "Debounce Limit"; inc "Debounce Increment"; dec "Debounce Decrement"; default "Default Value"; hi "Range High"; lo "Range Low"
  Subsys VINP_EDUSynchPosnPWMKDC_pct : inp_lib/valid_sat_ovrd  SystemSampleTime=-1  cal_ovrdflg=KINP_EDUSynchPosnPWMKDC_pct_ovrdflg  cal_ovrdval=KINP_EDUSynchPosnPWMKDC_pct_ovrdval  lim=KINP_ValidCheck_EDUSynchPosnPWMKDC_lim  inc=KINP_ValidCheck_EDUSynchPosnPWMKDC_inc  dec=KINP_ValidCheck_EDUSynchPosnPWMKDC_dec  default=KINP_EDUSynchPosnPWMKDCDefault_pct  hi=KINP_EDUSynchPosnPWMKDC_pct_UpperLimit  lo=KINP_EDUSynchPosnPWMKDC_pct_LowerLimit
  BINP_HardwireInputs : Outport  OutDataType=sfix(16)  OutScaling=2^0
  wires:
  [BSRV_In_ovrdflgs] -> Bus Selector29/1
  [BSRV_In_ovrdvals] -> Bus Selector28/1
  [BSRV_In_ovrdflgs] -> Bus Selector23/1
  [BSRV_In_ovrdvals] -> Bus Selector22/1
  BSRV_In_ovrdflgs/1 -> [BSRV_In_ovrdflgs]
  BSRV_In_ovrdvals/1 -> [BSRV_In_ovrdvals]
  [BSRV_In_ovrdflgs] -> Bus Selector18/1
  [BSRV_In_ovrdvals] -> Bus Selector17/1
  BHAL_outputs/1 -> Bus Selector43/1, Bus Selector30/1, Bus Selector50/1, Bus Selector19/1, Bus Selector41/1, Bus Selector24/1
  Bus Creator1/1 -> BINP_HardwireInputs/1  "BINP_HardwireInputs"
  Bus Selector24/1 -> Subsys VINP_EDUOutputShaftSpdRaw_rpm/1  "<VHAL_EDUOutputShaftSpdRawIn_rpm>"
  Bus Selector41/1 -> Subsys VINP_EDUOutputShaftSpdRaw_rpm/2  "<VHAL_EDUOutputShaftSpdRawValidIn_flg>"
  Bus Selector23/1 -> Subsys VINP_EDUOutputShaftSpdRaw_rpm/3  "<VSRV_EDUOutputShaftSpdRawIn_rpm_ovrdflg>"
  Bus Selector22/1 -> Subsys VINP_EDUOutputShaftSpdRaw_rpm/4  "<VSRV_EDUOutputShaftSpdRawIn_rpm_ovrdval>"
  Subsys VINP_EDUOutputShaftSpdRaw_rpm/1 -> Bus Creator1/1  "VINP_EDUOutputShaftSpdRaw_rpm"
  Subsys VINP_EDUOutputShaftSpdRaw_rpm/2 -> Bus Creator1/2  "VINP_EDUOutputShaftSpdRawValid_flg"
  Bus Selector19/1 -> Subsys VINP_EDUSynchPosnPWMKDC_pct/1  "<VHAL_EDUSynchPosnPWMKDCIn_pct>"
  Bus Selector50/1 -> Subsys VINP_EDUSynchPosnPWMKDC_pct/2  "<VHAL_EDUSynchPosnPWMKDCValidIn_flg>"
  Bus Selector18/1 -> Subsys VINP_EDUSynchPosnPWMKDC_pct/3  "<VSRV_EDUSynchPosnPWMKDCIn_pct_ovrdflg>"
  Bus Selector17/1 -> Subsys VINP_EDUSynchPosnPWMKDC_pct/4  "<VSRV_EDUSynchPosnPWMKDCIn_pct_ovrdval>"
  Subsys VINP_EDUSynchPosnPWMKDC_pct/1 -> Bus Creator1/3  "VINP_EDUSynchPosnPWMKDC_pct"
  Subsys VINP_EDUSynchPosnPWMKDC_pct/2 -> Bus Creator1/4  "VINP_EDUSynchPosnPWMKDCValid_flg"
  Bus Selector30/1 -> Subsys VINP_EDUSynchPosnPWMDC_pct/1(SigIn)  "<VHAL_EDUSynchPosnPWMDCIn_pct>"
  Subsys VINP_EDUSynchPosnPWMDC_pct/1(SigOut) -> Bus Creator1/5  "VINP_EDUSynchPosnPWMDC_pct"
  Subsys VINP_EDUSynchPosnPWMDC_pct/2(SigValid) -> Bus Creator1/6  "VINP_EDUSynchPosnPWMDCValid_flg"
  Bus Selector43/1 -> Subsys VINP_EDUSynchPosnPWMDC_pct/2(SigValidRaw)  "<VHAL_EDUSynchPosnPWMDCValidIn_flg>"
  Bus Selector29/1 -> Subsys VINP_EDUSynchPosnPWMDC_pct/3(srv_ovrdflg)  "<VSRV_EDUSynchPosnPWMDCIn_pct_ovrdflg>"
  Bus Selector28/1 -> Subsys VINP_EDUSynchPosnPWMDC_pct/4(srv_ovrdval)  "<VSRV_EDUSynchPosnPWMDCIn_pct_ovrdval>"

== system inp/INP/Pre-Process/BINP_ouputs_100ms ==
  trig_sig_chk : Inport  OutDataType=sfix(16)  OutScaling=2^0
  VINP_VehSpd_kph : Inport  Port=2  OutDataType=sfix(16)  OutScaling=2^0
  BINP_rawoutputs_100ms : Inport  Port=3  OutDataType=sfix(16)  OutScaling=2^0
  Bus Selector1 : BusSelector  OutputSignals=BINP_SMU_HSC_FrP06.VINP_BonnetOpenRaw_flg,BINP_SMU_HSC_FrP06.VINP_BonnetOpenRawValid_flg
  Outputs_100ms : Subsystem
  Signal Process : Subsystem
      settings: RTWSystemCode=Inline
  BINP_outputs_100ms : Outport  OutDataType=sfix(16)  OutScaling=2^0
  wires:
  Outputs_100ms/1(BINP_outputs_100ms) -> BINP_outputs_100ms/1
  Signal Process/1(VINP_BonnetOpen_flg) -> Outputs_100ms/1(VINP_BonnetOpen_flg)
  Bus Selector1/2 -> Signal Process/3(VINP_BonnetOpenRawValid_flg)  "<VINP_BonnetOpenRawValid_flg>"
  Bus Selector1/1 -> Signal Process/2(VINP_BonnetOpenRaw_flg)  "<VINP_BonnetOpenRaw_flg>"
  VINP_VehSpd_kph/1 -> Signal Process/1(VINP_VehSpd_kph)
  trig_sig_chk/1 -> Signal Process/Trigger
  BINP_rawoutputs_100ms/1 -> Outputs_100ms/2(BINP_rawoutputs_100ms), Bus Selector1/1

== system inp/INP/Pre-Process/BINP_ouputs_10ms ==
  trig_sig_chk_10ms : Inport  OutDataType=sfix(16)  OutScaling=2^0
  VINP_VehSpd_kph : Inport  Port=2  OutDataType=sfix(16)  OutScaling=2^0
  VINP_VehSpdValid_flg : Inport  Port=3  OutDataType=sfix(16)  OutScaling=2^0
  BINP_rawoutputs_10ms : Inport  Port=4  OutDataType=sfix(16)  OutScaling=2^0
  VDSM_SngAccPedInvldFlt_flg : Inport  Port=5  OutDataType=sfix(16)  OutScaling=2^0
  Signal Process : Subsystem
      settings: RTWSystemCode=Inline
  outputs_10ms : Subsystem
  BINP_outputs_10ms : Outport  OutDataType=sfix(16)  OutScaling=2^0
  wires:
  VDSM_SngAccPedInvldFlt_flg/1 -> Signal Process/2(VDSM_SngAccPedInvldFlt_flg)
  Signal Process/4(VINP_ISGSpdValid_flg) -> outputs_10ms/7(VINP_ISGSpdValid_flg)
  Signal Process/2(VINP_EngSpdValid_flg) -> outputs_10ms/5(VINP_EngSpdValid_flg)
  Signal Process/3(VINP_ISGSpd_rpm) -> outputs_10ms/6(VINP_ISGSpd_rpm)
  Signal Process/1(VINP_EngSpd_rpm) -> outputs_10ms/4(VINP_EngSpd_rpm)
  trig_sig_chk_10ms/1 -> Signal Process/Trigger
  BINP_rawoutputs_10ms/1 -> Signal Process/1(BINP_rawoutputs_10ms), outputs_10ms/1(BINP_rawoutputs_10ms)
  VINP_VehSpdValid_flg/1 -> outputs_10ms/3(VINP_VehSpdValid_flg)
  VINP_VehSpd_kph/1 -> outputs_10ms/2(VINP_VehSpd_kph)
  outputs_10ms/1(BINP_outputs_10ms) -> BINP_outputs_10ms/1
  Signal Process/5(VINP_AccelPedalPosn_pct) -> outputs_10ms/8(VINP_AccelPedalPosn_pct)

== system inp/INP/Pre-Process/BINP_ouputs_5ms ==
  trig_sig_chk : Inport  OutDataType=sfix(16)  OutScaling=2^0
  BINP_rawoutputs_5ms : Inport  Port=2  OutDataType=sfix(16)  OutScaling=2^0
  BINP_rawoutputs_10ms : Inport  Port=3  OutDataType=sfix(16)  OutScaling=2^0
  Bus Selector1 : BusSelector  OutputSignals=BINP_ABS_DSC_HSC_FrP00.VINP_VehSpdRawABS_kph,BINP_ABS_DSC_HSC_FrP00.VINP_VehSpdRawValid_flg,BINP_TC_HSC2_FrP01.VINP_TMSpd_rpm
  Bus Selector2 : BusSelector  OutputSignals=BINP_HardwireInputs.VINP_EDUSynchPosnPWMKDC_pct,BINP_HardwireInputs.VINP_EDUSynchPosnPWMKDCValid_flg,BINP_HardwireInputs.VINP_EDUSynchPosnPWMDC_pct,BINP_HardwireInputs.VINP_EDUSynchPosnPWMDCValid_flg,BINP_HardwireInputs.VINP_EDUOutputShaftSpdRaw_rpm,BINP_HardwireInputs.VINP_EDUOutputShaftSpdRawValid_flg
  Outputs_5ms : Subsystem
  Signal Process : Subsystem
      settings: RTWSystemCode=Inline
  BINP_outputs_5ms : Outport  OutDataType=sfix(16)  OutScaling=2^0
  VINP_VehSpd_kph : Outport  Port=2  OutDataType=sfix(16)  OutScaling=2^0
  VINP_VehSpdValid_flg : Outport  Port=3  OutDataType=sfix(16)  OutScaling=2^0
  wires:
  Bus Selector1/3 -> Signal Process/9(VINP_TMSpd_rpm)  "<VINP_TMSpd_rpm>"
  Signal Process/6(VINP_VehSpdValid_flg) -> VINP_VehSpdValid_flg/1
  Signal Process/5(VINP_VehSpd_kph) -> VINP_VehSpd_kph/1
  trig_sig_chk/1 -> Signal Process/Trigger
  Outputs_5ms/1(BINP_outputs_5ms) -> BINP_outputs_5ms/1  "BINP_outputs_5ms"
  Signal Process/1(VINP_EDUOutputShaftSpd_rpm) -> Outputs_5ms/2(VINP_EDUOutputShaftSpd_rpm)
  Signal Process/2(VINP_EDUOutputShaftSpdValid_flg) -> Outputs_5ms/3(VINP_EDUOutputShaftSpdRawValid_flg)
  Signal Process/3(VINP_EDUSynchPosn_mm) -> Outputs_5ms/4(VINP_EDUSynchPosn_mm)
  Signal Process/4(VINP_EDUSynchPosnValid_flg) -> Outputs_5ms/5(VINP_EDUSynchPosnValid_flg)
  BINP_rawoutputs_10ms/1 -> Bus Selector1/1
  Bus Selector2/6 -> Signal Process/6(VINP_EDUOutputShaftSpdRawValid_flg)  "<VINP_EDUOutputShaftSpdRawValid_flg>"
  Bus Selector2/5 -> Signal Process/5(VINP_EDUOutputShaftSpdRaw_rpm)  "<VINP_EDUOutputShaftSpdRaw_rpm>"
  Bus Selector2/4 -> Signal Process/4(VINP_EDUSynchPosnPWMDCValid_flg)  "<VINP_EDUSynchPosnPWMDCValid_flg>"
  Bus Selector2/3 -> Signal Process/3(VINP_EDUSynchPosnPWMDC_pct)  "<VINP_EDUSynchPosnPWMDC_pct>"
  Bus Selector2/2 -> Signal Process/2(VINP_EDUSynchPosnPWMKDCValid_flg)  "<VINP_EDUSynchPosnPWMKDCValid_flg>"
  Bus Selector2/1 -> Signal Process/1(VINP_EDUSynchPosnPWMKDC_pct)  "<VINP_EDUSynchPosnPWMKDC_pct>"
  BINP_rawoutputs_5ms/1 -> Outputs_5ms/1(BINP_rawoutputs_5ms), Bus Selector2/1
  Bus Selector1/1 -> Signal Process/7(VINP_VehSpdRawABS_kph)  "<VINP_VehSpdRawABS_kph>"
  Bus Selector1/2 -> Signal Process/8(VINP_VehSpdRawValid_flg)  "<VINP_VehSpdRawValid_flg>"

== system inp/INP/Version_Control/Submit ==

== system inp/INP/INP_100MS/HW_HCU_100ms/filter ==
  VINP_EDUCoolantTempRaw_C : Inport  OutDataType=sfix(16)  OutScaling=2^0
  Constant : Constant  Value=0.1  OutDataTypeMode=single  OutDataType=fixdt(1, 16)  OutScaling=2^0  OutDataTypeStr=single
  Constant1 : Constant  Value=KINP_EDUCoolantTempFilTm_s  OutDataTypeMode=single  OutDataType=fixdt(1, 16)  OutScaling=2^0  OutDataTypeStr=single
  First_Order_Filter : hcu_lib/First_Order_Filter  SystemSampleTime=-1
  VINP_EDUCoolantTemp_C : Outport  OutDataType=sfix(16)  OutScaling=2^0
  wires:
  Constant1/1 -> First_Order_Filter/2
  Constant/1 -> First_Order_Filter/3
  First_Order_Filter/1 -> VINP_EDUCoolantTemp_C/1
  VINP_EDUCoolantTempRaw_C/1 -> First_Order_Filter/1

== system inp/INP/INP_100MS/HW_HCU_100ms/filter1 ==
  VINP_EDUOilTempRaw_C : Inport  OutDataType=sfix(16)  OutScaling=2^0
  Constant : Constant  Value=0.1  OutDataTypeMode=single  OutDataType=fixdt(1, 16)  OutScaling=2^0  OutDataTypeStr=single
  Constant1 : Constant  Value=KINP_EDUOilTempFilTm_s  OutDataTypeMode=single  OutDataType=fixdt(1, 16)  OutScaling=2^0  OutDataTypeStr=single
  First_Order_Filter : hcu_lib/First_Order_Filter  SystemSampleTime=-1
  VINP_EDUOilTemp_C : Outport  OutDataType=sfix(16)  OutScaling=2^0
  wires:
  Constant/1 -> First_Order_Filter/3
  Constant1/1 -> First_Order_Filter/2
  First_Order_Filter/1 -> VINP_EDUOilTemp_C/1
  VINP_EDUOilTempRaw_C/1 -> First_Order_Filter/1
